simulink library "Ramp_Library_R2017b"  (R2017b)
settings: Solver=VariableStepAuto  StartTime=0.0  StopTime=10.0  RelTol=1e-3
libraries: simulink x52
(part 1 of 2)
Description:
  | VLS Standard Library
  | Version: 1.0.0
settings Model: Creator=mchawa  LastModifiedBy=mchawa

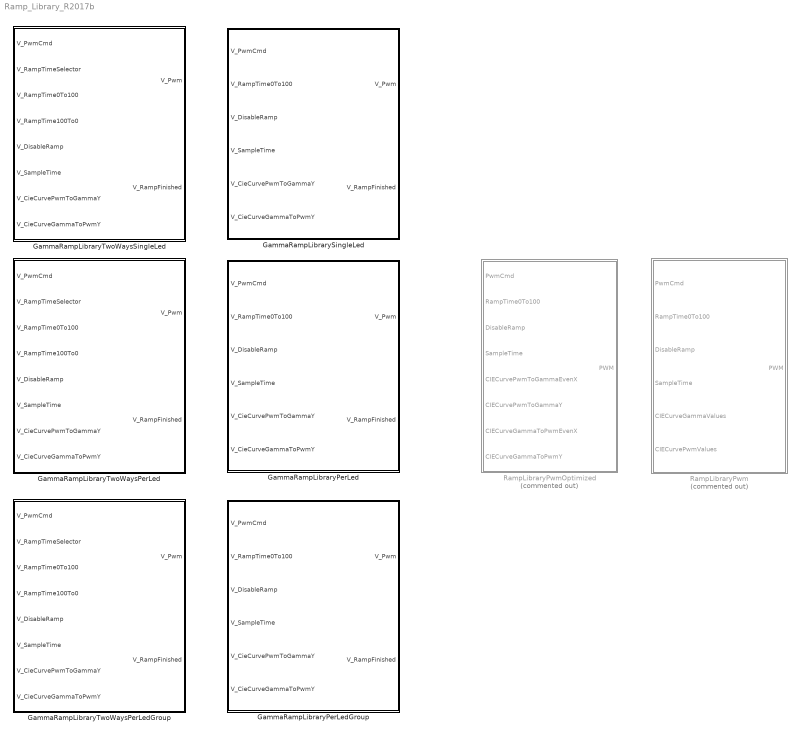
== system Ramp_Library_R2017b ==
  GammaRampLibraryPerLed : Subsystem  Description=|
      | This library performs ramp function taking CIE curves which are evenly distributed.
      | It performs the ramp linearly on the Gamma Curve.
  GammaRampLibraryPerLedGroup : Subsystem  Description=|
      | This library performs ramp function taking CIE curves which are evenly distributed.
      | It performs the ramp linearly on the Gamma Curve.
  GammaRampLibrarySingleLed : Subsystem  Description=|
      | This library performs ramp function taking CIE curves which are evenly distributed.
      | It performs the ramp linearly on the Gamma Curve.
  GammaRampLibraryTwoWaysPerLed : Subsystem  Description=|
      | This library performs ramp function taking CIE curves which are evenly distributed.
      | It performs the ramp linearly on the Gamma Curve.
  GammaRampLibraryTwoWaysPerLedGroup : Subsystem  Description=|
      | This library performs ramp function taking CIE curves which are evenly distributed.
      | It performs the ramp linearly on the Gamma Curve.
  GammaRampLibraryTwoWaysSingleLed : Subsystem  Description=|
      | This library performs ramp function taking CIE curves which are evenly distributed.
      | It performs the ramp linearly on the Gamma Curve.
  RampLibraryPwm : Subsystem  Description=|  Commented=on
      | This library performs ramp function taking CIE curves.
      | It performs the ramp linearly on the Pwm Curve.
  RampLibraryPwmOptimized : Subsystem  Description=|  Commented=on
      | This library performs ramp function taking CIE curves which are evenly distributed.
      | It performs the ramp linearly on the Pwm Curve.

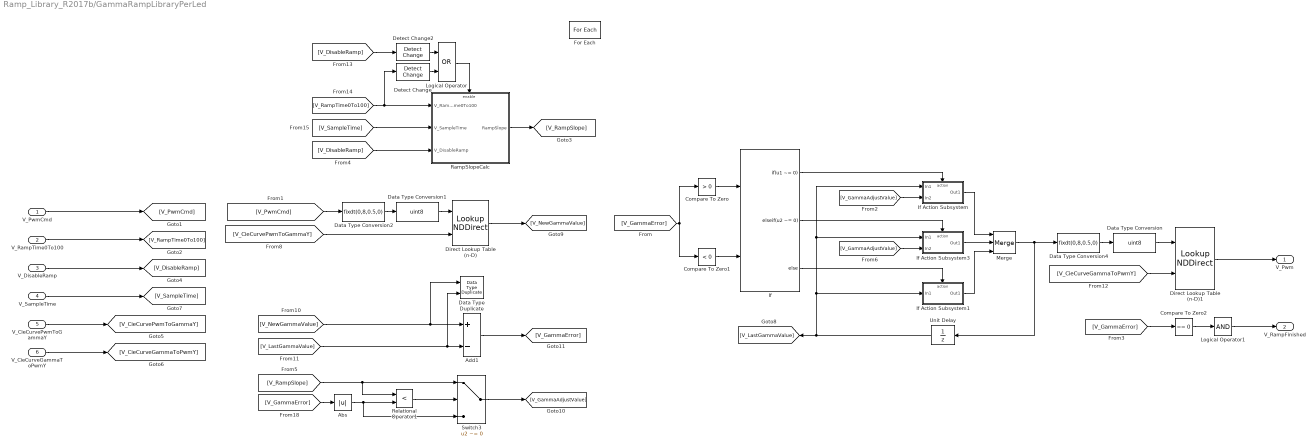
== system Ramp_Library_R2017b/GammaRampLibraryPerLed ==
  V_PwmCmd : Inport  Partition=on  PartitionDimension=1  PartitionWidth=1  PartitionOffset=0
  V_RampTime0To100 : Inport  Port=2  Partition=on  PartitionDimension=1  PartitionWidth=1  PartitionOffset=0
  V_DisableRamp : Inport  Port=3
  V_SampleTime : Inport  Port=4
  V_CieCurvePwmToGammaY : Inport  Port=5
  V_CieCurveGammaToPwmY : Inport  Port=6
  Abs : Abs
  Add1 : Sum  Inputs=+-  OutMin=-100  OutMax=100  OutDataTypeStr=fixdt(1,16,0.01,0)
  Compare To Zero : simulink/Logic and Bit Operations/Compare To Zero  relop=>  OutDataTypeStr=boolean
  Compare To Zero1 : simulink/Logic and Bit Operations/Compare To Zero  relop=<  OutDataTypeStr=boolean
  Compare To Zero2 : simulink/Logic and Bit Operations/Compare To Zero  relop===  OutDataTypeStr=boolean
  Data Type Duplicate : DataTypeDuplicate
  Data Type Conversion : DataTypeConversion  OutDataTypeStr=uint8  ConvertRealWorld=Stored Integer (SI)
  Data Type Conversion1 : DataTypeConversion  OutDataTypeStr=uint8  ConvertRealWorld=Stored Integer (SI)
  Data Type Conversion2 : DataTypeConversion  OutDataTypeStr=fixdt(0,8,0.5,0)  RndMeth=Round
  Data Type Conversion4 : DataTypeConversion  OutDataTypeStr=fixdt(0,8,0.5,0)  RndMeth=Round
  Detect Change : simulink/Logic and Bit Operations/Detect Change  vinit=0  OutDataTypeStr=boolean
  Detect Change2 : simulink/Logic and Bit Operations/Detect Change  vinit=0  OutDataTypeStr=boolean
  Direct Lookup Table (n-D) : LookupNDDirect  NumberOfTableDimensions=1  TableIsInput=on
  Direct Lookup Table (n-D)1 : LookupNDDirect  NumberOfTableDimensions=1  TableIsInput=on
  For Each : ForEach  DisableCoverage=on  IndexMode=One-based
  If : If  NumInputs=2  IfExpression=u1 ~= 0  ElseIfExpressions=u2 ~= 0
  If Action Subsystem : Subsystem  TreatAsAtomicUnit=on
  If Action Subsystem1 : Subsystem  TreatAsAtomicUnit=on
  If Action Subsystem3 : Subsystem  TreatAsAtomicUnit=on
  Logical Operator : Logic  Operator=OR  AllPortsSameDT=off  OutDataTypeStr=boolean
  Logical Operator1 : Logic  Inputs=1  AllPortsSameDT=off  OutDataTypeStr=boolean
  Merge : Merge  Inputs=3
  RampSlopeCalc : Subsystem  TreatAsAtomicUnit=on
  Relational Operator1 : RelationalOperator  Operator=<  OutDataTypeStr=boolean  RndMeth=Simplest
  Switch3 : Switch  Criteria=u2 ~= 0  OutDataTypeStr=Inherit: Inherit via back propagation
  Unit Delay : UnitDelay  SampleTime=-1
  V_Pwm : Outport  ConcatenationDimension=1
  V_RampFinished : Outport  Port=2  ConcatenationDimension=1
  wires:
  [V_CieCurveGammaToPwmY] -> Direct Lookup Table (n-D)1/2
  [V_GammaError] -> Compare To Zero1/1, Compare To Zero/1
  [V_NewGammaValue] -> Add1/1, Data Type Duplicate/1
  If Action Subsystem/1(Out1) -> Merge/1
  If Action Subsystem1/1(Out1) -> Merge/3
  Abs/1 -> Switch3/3, Relational Operator1/2
  V_PwmCmd/1 -> [V_PwmCmd]
  V_CieCurvePwmToGammaY/1 -> [V_CieCurvePwmToGammaY]
  [V_GammaError] -> Abs/1
  [V_PwmCmd] -> Data Type Conversion2/1
  Data Type Conversion/1 -> Direct Lookup Table (n-D)1/1
  Detect Change/1 -> Logical Operator/2
  Data Type Conversion4/1 -> Data Type Conversion/1
  [V_CieCurvePwmToGammaY] -> Direct Lookup Table (n-D)/2
  Switch3/1 -> [V_GammaAdjustValue]
  V_SampleTime/1 -> [V_SampleTime]
  Relational Operator1/1 -> Switch3/2
  V_RampTime0To100/1 -> [V_RampTime0To100]
  Compare To Zero/1 -> If/1
  If/3 -> If Action Subsystem1/Action
  Unit Delay/1 -> If Action Subsystem/1(In1), If Action Subsystem3/1(In1), If Action Subsystem1/1(In1), [V_LastGammaValue]
  [V_GammaAdjustValue] -> If Action Subsystem/2(In2)
  [V_RampSlope] -> Switch3/1, Relational Operator1/1
  [V_RampTime0To100] -> Detect Change/1, RampSlopeCalc/1(V_RampTime0To100)
  If/2 -> If Action Subsystem3/Action
  V_DisableRamp/1 -> [V_DisableRamp]
  Data Type Conversion1/1 -> Direct Lookup Table (n-D)/1
  [V_DisableRamp] -> RampSlopeCalc/3(V_DisableRamp)
  [V_LastGammaValue] -> Add1/2, Data Type Duplicate/2
  Add1/1 -> [V_GammaError]
  Logical Operator/1 -> RampSlopeCalc/Enable
  Merge/1 -> Data Type Conversion4/1, Unit Delay/1
  Direct Lookup Table (n-D)/1 -> [V_NewGammaValue]
  [V_SampleTime] -> RampSlopeCalc/2(V_SampleTime)
  Direct Lookup Table (n-D)1/1 -> V_Pwm/1
  V_CieCurveGammaToPwmY/1 -> [V_CieCurveGammaToPwmY]
  [V_DisableRamp] -> Detect Change2/1
  Compare To Zero1/1 -> If/2
  Data Type Conversion2/1 -> Data Type Conversion1/1
  If Action Subsystem3/1(Out1) -> Merge/2
  [V_GammaAdjustValue] -> If Action Subsystem3/2(In2)
  RampSlopeCalc/1(RampSlope) -> [V_RampSlope]
  Detect Change2/1 -> Logical Operator/1
  If/1 -> If Action Subsystem/Action
  [V_GammaError] -> Compare To Zero2/1
  Compare To Zero2/1 -> Logical Operator1/1
  Logical Operator1/1 -> V_RampFinished/1

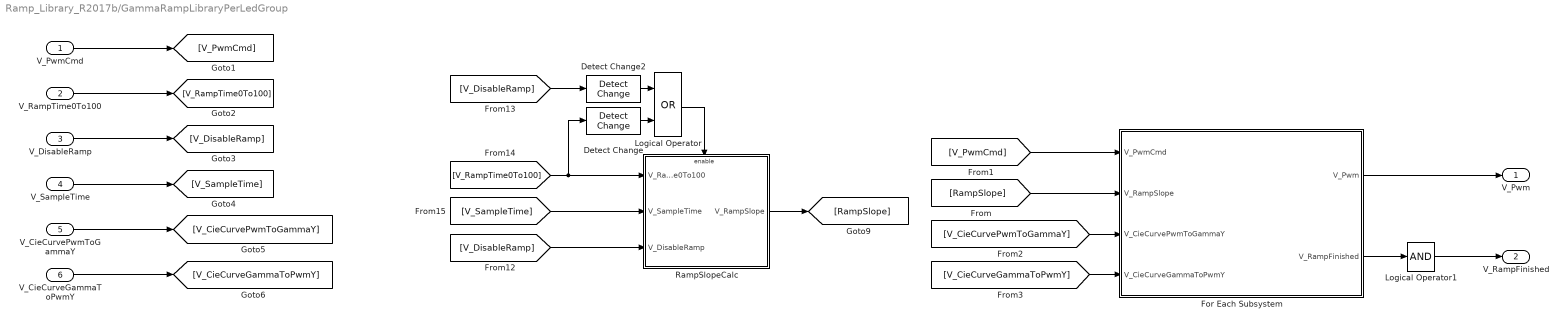
== system Ramp_Library_R2017b/GammaRampLibraryPerLedGroup ==
  V_PwmCmd : Inport
  V_RampTime0To100 : Inport  Port=2
  V_DisableRamp : Inport  Port=3
  V_SampleTime : Inport  Port=4
  V_CieCurvePwmToGammaY : Inport  Port=5
  V_CieCurveGammaToPwmY : Inport  Port=6
  Detect Change : simulink/Logic and Bit Operations/Detect Change  vinit=0  OutDataTypeStr=boolean
  Detect Change2 : simulink/Logic and Bit Operations/Detect Change  vinit=0  OutDataTypeStr=boolean
  For Each Subsystem : Subsystem  TreatAsAtomicUnit=on
  Logical Operator : Logic  Operator=OR  AllPortsSameDT=off  OutDataTypeStr=boolean
  Logical Operator1 : Logic  Inputs=1  AllPortsSameDT=off  OutDataTypeStr=boolean
  RampSlopeCalc : Subsystem  TreatAsAtomicUnit=on
  V_Pwm : Outport
  V_RampFinished : Outport  Port=2
  wires:
  V_PwmCmd/1 -> [V_PwmCmd]
  V_RampTime0To100/1 -> [V_RampTime0To100]
  V_DisableRamp/1 -> [V_DisableRamp]
  V_SampleTime/1 -> [V_SampleTime]
  V_CieCurvePwmToGammaY/1 -> [V_CieCurvePwmToGammaY]
  V_CieCurveGammaToPwmY/1 -> [V_CieCurveGammaToPwmY]
  RampSlopeCalc/1(V_RampSlope) -> [RampSlope]
  Logical Operator/1 -> RampSlopeCalc/Enable
  Detect Change/1 -> Logical Operator/2
  [V_DisableRamp] -> Detect Change2/1
  [V_DisableRamp] -> RampSlopeCalc/3(V_DisableRamp)
  [V_SampleTime] -> RampSlopeCalc/2(V_SampleTime)
  [V_RampTime0To100] -> RampSlopeCalc/1(V_RampTime0To100), Detect Change/1
  Detect Change2/1 -> Logical Operator/1
  [RampSlope] -> For Each Subsystem/2(V_RampSlope)
  [V_PwmCmd] -> For Each Subsystem/1(V_PwmCmd)
  [V_CieCurvePwmToGammaY] -> For Each Subsystem/3(V_CieCurvePwmToGammaY)
  For Each Subsystem/1(V_Pwm) -> V_Pwm/1
  [V_CieCurveGammaToPwmY] -> For Each Subsystem/4(V_CieCurveGammaToPwmY)
  For Each Subsystem/2(V_RampFinished) -> Logical Operator1/1
  Logical Operator1/1 -> V_RampFinished/1

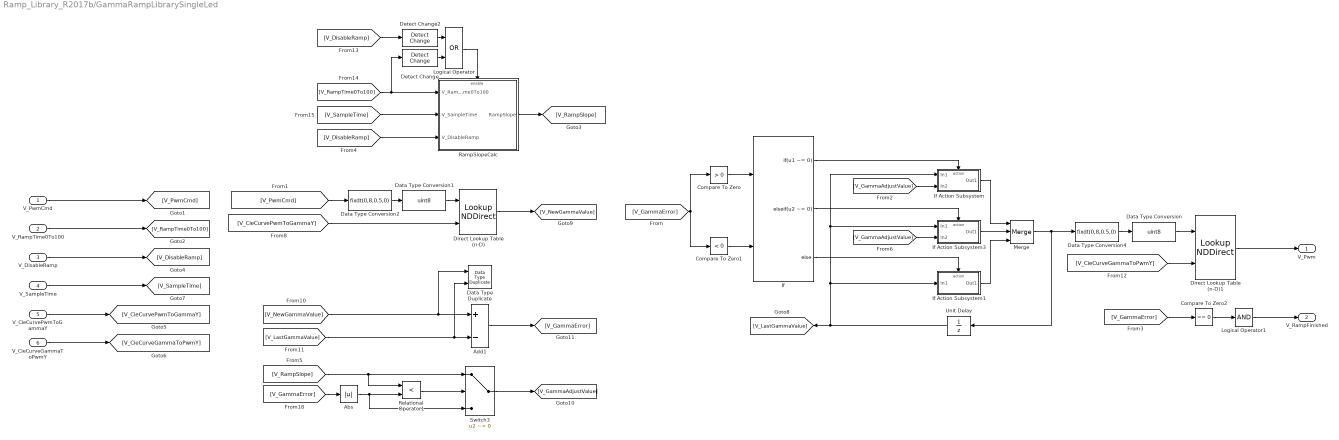
== system Ramp_Library_R2017b/GammaRampLibrarySingleLed ==
  V_PwmCmd : Inport
  V_RampTime0To100 : Inport  Port=2
  V_DisableRamp : Inport  Port=3
  V_SampleTime : Inport  Port=4
  V_CieCurvePwmToGammaY : Inport  Port=5
  V_CieCurveGammaToPwmY : Inport  Port=6
  Abs : Abs
  Add1 : Sum  Inputs=+-  OutMin=-100  OutMax=100  OutDataTypeStr=fixdt(1,16,0.01,0)
  Compare To Zero : simulink/Logic and Bit Operations/Compare To Zero  relop=>  OutDataTypeStr=boolean
  Compare To Zero1 : simulink/Logic and Bit Operations/Compare To Zero  relop=<  OutDataTypeStr=boolean
  Compare To Zero2 : simulink/Logic and Bit Operations/Compare To Zero  relop===  OutDataTypeStr=boolean
  Data Type Duplicate : DataTypeDuplicate
  Data Type Conversion : DataTypeConversion  OutDataTypeStr=uint8  ConvertRealWorld=Stored Integer (SI)
  Data Type Conversion1 : DataTypeConversion  OutDataTypeStr=uint8  ConvertRealWorld=Stored Integer (SI)
  Data Type Conversion2 : DataTypeConversion  OutDataTypeStr=fixdt(0,8,0.5,0)  RndMeth=Round
  Data Type Conversion4 : DataTypeConversion  OutDataTypeStr=fixdt(0,8,0.5,0)  RndMeth=Round
  Detect Change : simulink/Logic and Bit Operations/Detect Change  vinit=0  OutDataTypeStr=boolean
  Detect Change2 : simulink/Logic and Bit Operations/Detect Change  vinit=0  OutDataTypeStr=boolean
  Direct Lookup Table (n-D) : LookupNDDirect  NumberOfTableDimensions=1  TableIsInput=on
  Direct Lookup Table (n-D)1 : LookupNDDirect  NumberOfTableDimensions=1  TableIsInput=on
  If : If  NumInputs=2  IfExpression=u1 ~= 0  ElseIfExpressions=u2 ~= 0
  If Action Subsystem : Subsystem  TreatAsAtomicUnit=on
  If Action Subsystem1 : Subsystem  TreatAsAtomicUnit=on
  If Action Subsystem3 : Subsystem  TreatAsAtomicUnit=on
  Logical Operator : Logic  Operator=OR  AllPortsSameDT=off  OutDataTypeStr=boolean
  Logical Operator1 : Logic  Inputs=1  AllPortsSameDT=off  OutDataTypeStr=boolean
  Merge : Merge  Inputs=3
  RampSlopeCalc : Subsystem  TreatAsAtomicUnit=on
  Relational Operator1 : RelationalOperator  Operator=<  OutDataTypeStr=boolean  RndMeth=Simplest
  Switch3 : Switch  Criteria=u2 ~= 0  OutDataTypeStr=Inherit: Inherit via back propagation
  Unit Delay : UnitDelay  SampleTime=-1
  V_Pwm : Outport
  V_RampFinished : Outport  Port=2
  wires:
  Logical Operator1/1 -> V_RampFinished/1
  Compare To Zero2/1 -> Logical Operator1/1
  [V_GammaError] -> Compare To Zero2/1
  If/1 -> If Action Subsystem/Action
  Detect Change2/1 -> Logical Operator/1
  RampSlopeCalc/1(RampSlope) -> [V_RampSlope]
  [V_GammaAdjustValue] -> If Action Subsystem3/2(In2)
  If Action Subsystem3/1(Out1) -> Merge/2
  Data Type Conversion2/1 -> Data Type Conversion1/1
  Compare To Zero1/1 -> If/2
  [V_DisableRamp] -> Detect Change2/1
  V_CieCurveGammaToPwmY/1 -> [V_CieCurveGammaToPwmY]
  Direct Lookup Table (n-D)1/1 -> V_Pwm/1
  [V_SampleTime] -> RampSlopeCalc/2(V_SampleTime)
  Direct Lookup Table (n-D)/1 -> [V_NewGammaValue]
  Merge/1 -> Unit Delay/1, Data Type Conversion4/1
  Logical Operator/1 -> RampSlopeCalc/Enable
  Add1/1 -> [V_GammaError]
  [V_LastGammaValue] -> Data Type Duplicate/2, Add1/2
  [V_DisableRamp] -> RampSlopeCalc/3(V_DisableRamp)
  Data Type Conversion1/1 -> Direct Lookup Table (n-D)/1
  V_DisableRamp/1 -> [V_DisableRamp]
  If/2 -> If Action Subsystem3/Action
  [V_RampTime0To100] -> RampSlopeCalc/1(V_RampTime0To100), Detect Change/1
  [V_RampSlope] -> Relational Operator1/1, Switch3/1
  [V_GammaAdjustValue] -> If Action Subsystem/2(In2)
  Unit Delay/1 -> [V_LastGammaValue], If Action Subsystem1/1(In1), If Action Subsystem3/1(In1), If Action Subsystem/1(In1)
  If/3 -> If Action Subsystem1/Action
  Compare To Zero/1 -> If/1
  V_RampTime0To100/1 -> [V_RampTime0To100]
  Relational Operator1/1 -> Switch3/2
  V_SampleTime/1 -> [V_SampleTime]
  Switch3/1 -> [V_GammaAdjustValue]
  [V_CieCurvePwmToGammaY] -> Direct Lookup Table (n-D)/2
  Data Type Conversion4/1 -> Data Type Conversion/1
  Detect Change/1 -> Logical Operator/2
  Data Type Conversion/1 -> Direct Lookup Table (n-D)1/1
  [V_PwmCmd] -> Data Type Conversion2/1
  [V_GammaError] -> Abs/1
  V_CieCurvePwmToGammaY/1 -> [V_CieCurvePwmToGammaY]
  V_PwmCmd/1 -> [V_PwmCmd]
  Abs/1 -> Relational Operator1/2, Switch3/3
  If Action Subsystem1/1(Out1) -> Merge/3
  If Action Subsystem/1(Out1) -> Merge/1
  [V_NewGammaValue] -> Data Type Duplicate/1, Add1/1
  [V_GammaError] -> Compare To Zero/1, Compare To Zero1/1
  [V_CieCurveGammaToPwmY] -> Direct Lookup Table (n-D)1/2

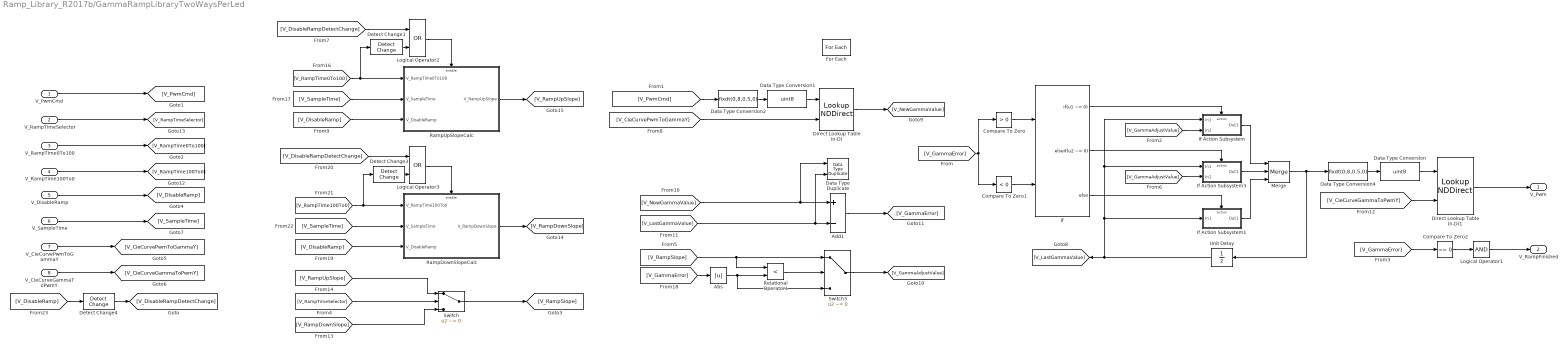
== system Ramp_Library_R2017b/GammaRampLibraryTwoWaysPerLed ==
  V_PwmCmd : Inport  Partition=on  PartitionDimension=1  PartitionWidth=1  PartitionOffset=0
  V_RampTimeSelector : Inport  Port=2  Partition=on  PartitionDimension=1  PartitionWidth=1  PartitionOffset=0
  V_RampTime0To100 : Inport  Port=3  Partition=on  PartitionDimension=1  PartitionWidth=1  PartitionOffset=0
  V_RampTime100To0 : Inport  Port=4  Partition=on  PartitionDimension=1  PartitionWidth=1  PartitionOffset=0
  V_DisableRamp : Inport  Port=5
  V_SampleTime : Inport  Port=6
  V_CieCurvePwmToGammaY : Inport  Port=7
  V_CieCurveGammaToPwmY : Inport  Port=8
  Abs : Abs
  Add1 : Sum  Inputs=+-  OutMin=-100  OutMax=100  OutDataTypeStr=fixdt(1,16,0.01,0)
  Compare To Zero : simulink/Logic and Bit Operations/Compare To Zero  relop=>  OutDataTypeStr=boolean
  Compare To Zero1 : simulink/Logic and Bit Operations/Compare To Zero  relop=<  OutDataTypeStr=boolean
  Compare To Zero2 : simulink/Logic and Bit Operations/Compare To Zero  relop===  OutDataTypeStr=boolean
  Data Type Duplicate : DataTypeDuplicate
  Data Type Conversion : DataTypeConversion  OutDataTypeStr=uint8  ConvertRealWorld=Stored Integer (SI)
  Data Type Conversion1 : DataTypeConversion  OutDataTypeStr=uint8  ConvertRealWorld=Stored Integer (SI)
  Data Type Conversion2 : DataTypeConversion  OutDataTypeStr=fixdt(0,8,0.5,0)  RndMeth=Round
  Data Type Conversion4 : DataTypeConversion  OutDataTypeStr=fixdt(0,8,0.5,0)  RndMeth=Round
  Detect Change1 : simulink/Logic and Bit Operations/Detect Change  vinit=0  OutDataTypeStr=boolean
  Detect Change3 : simulink/Logic and Bit Operations/Detect Change  vinit=0  OutDataTypeStr=boolean
  Detect Change4 : simulink/Logic and Bit Operations/Detect Change  vinit=0  OutDataTypeStr=boolean
  Direct Lookup Table (n-D) : LookupNDDirect  NumberOfTableDimensions=1  TableIsInput=on
  Direct Lookup Table (n-D)1 : LookupNDDirect  NumberOfTableDimensions=1  TableIsInput=on
  For Each : ForEach  DisableCoverage=on  IndexMode=One-based
  If : If  NumInputs=2  IfExpression=u1 ~= 0  ElseIfExpressions=u2 ~= 0
  If Action Subsystem : Subsystem  TreatAsAtomicUnit=on
  If Action Subsystem1 : Subsystem  TreatAsAtomicUnit=on
  If Action Subsystem3 : Subsystem  TreatAsAtomicUnit=on
  Logical Operator1 : Logic  Inputs=1  AllPortsSameDT=off  OutDataTypeStr=boolean
  Logical Operator2 : Logic  Operator=OR  AllPortsSameDT=off  OutDataTypeStr=boolean
  Logical Operator3 : Logic  Operator=OR  AllPortsSameDT=off  OutDataTypeStr=boolean
  Merge : Merge  Inputs=3
  RampDownSlopeCalc : Subsystem  TreatAsAtomicUnit=on
  RampUpSlopeCalc : Subsystem  TreatAsAtomicUnit=on
  Relational Operator1 : RelationalOperator  Operator=<  OutDataTypeStr=boolean  RndMeth=Simplest
  Switch : Switch  Criteria=u2 ~= 0
  Switch3 : Switch  Criteria=u2 ~= 0  OutDataTypeStr=Inherit: Inherit via back propagation
  Unit Delay : UnitDelay  SampleTime=-1
  V_Pwm : Outport  ConcatenationDimension=1
  V_RampFinished : Outport  Port=2  ConcatenationDimension=1
  wires:
  Logical Operator1/1 -> V_RampFinished/1
  Compare To Zero2/1 -> Logical Operator1/1
  [V_GammaError] -> Compare To Zero2/1
  If/1 -> If Action Subsystem/Action
  [V_GammaAdjustValue] -> If Action Subsystem3/2(In2)
  If Action Subsystem3/1(Out1) -> Merge/2
  Data Type Conversion2/1 -> Data Type Conversion1/1
  Compare To Zero1/1 -> If/2
  V_CieCurveGammaToPwmY/1 -> [V_CieCurveGammaToPwmY]
  Direct Lookup Table (n-D)1/1 -> V_Pwm/1
  Direct Lookup Table (n-D)/1 -> [V_NewGammaValue]
  Merge/1 -> Unit Delay/1, Data Type Conversion4/1
  Add1/1 -> [V_GammaError]
  [V_LastGammaValue] -> Data Type Duplicate/2, Add1/2
  Data Type Conversion1/1 -> Direct Lookup Table (n-D)/1
  V_DisableRamp/1 -> [V_DisableRamp]
  If/2 -> If Action Subsystem3/Action
  [V_RampSlope] -> Relational Operator1/1, Switch3/1
  [V_GammaAdjustValue] -> If Action Subsystem/2(In2)
  Unit Delay/1 -> [V_LastGammaValue], If Action Subsystem1/1(In1), If Action Subsystem3/1(In1), If Action Subsystem/1(In1)
  If/3 -> If Action Subsystem1/Action
  Compare To Zero/1 -> If/1
  V_RampTime0To100/1 -> [V_RampTime0To100]
  Relational Operator1/1 -> Switch3/2
  V_SampleTime/1 -> [V_SampleTime]
  Switch3/1 -> [V_GammaAdjustValue]
  [V_CieCurvePwmToGammaY] -> Direct Lookup Table (n-D)/2
  Data Type Conversion4/1 -> Data Type Conversion/1
  Data Type Conversion/1 -> Direct Lookup Table (n-D)1/1
  [V_PwmCmd] -> Data Type Conversion2/1
  [V_GammaError] -> Abs/1
  V_CieCurvePwmToGammaY/1 -> [V_CieCurvePwmToGammaY]
  V_PwmCmd/1 -> [V_PwmCmd]
  Abs/1 -> Relational Operator1/2, Switch3/3
  If Action Subsystem1/1(Out1) -> Merge/3
  If Action Subsystem/1(Out1) -> Merge/1
  [V_NewGammaValue] -> Data Type Duplicate/1, Add1/1
  [V_GammaError] -> Compare To Zero1/1, Compare To Zero/1
  [V_CieCurveGammaToPwmY] -> Direct Lookup Table (n-D)1/2
  V_RampTime100To0/1 -> [V_RampTime100To0]
  V_RampTimeSelector/1 -> [V_RampTimeSelector]
  Logical Operator2/1 -> RampUpSlopeCalc/Enable
  Detect Change3/1 -> Logical Operator3/2
  RampDownSlopeCalc/1(V_RampDownSlope) -> [V_RampDownSlope]
  [V_SampleTime] -> RampUpSlopeCalc/2(V_SampleTime)
  [V_DisableRampDetectChange] -> Logical Operator2/1
  [V_DisableRampDetectChange] -> Logical Operator3/1
  RampUpSlopeCalc/1(V_RampUpSlope) -> [V_RampUpSlope]
  Detect Change1/1 -> Logical Operator2/2
  [V_DisableRamp] -> RampDownSlopeCalc/3(V_DisableRamp)
  [V_RampTime100To0] -> RampDownSlopeCalc/1(V_RampTime100To0), Detect Change3/1
  [V_SampleTime] -> RampDownSlopeCalc/2(V_SampleTime)
  [V_DisableRamp] -> RampUpSlopeCalc/3(V_DisableRamp)
  Logical Operator3/1 -> RampDownSlopeCalc/Enable
  [V_RampTime0To100] -> Detect Change1/1, RampUpSlopeCalc/1(V_RampTime0To100)
  [V_DisableRamp] -> Detect Change4/1
  Detect Change4/1 -> [V_DisableRampDetectChange]
  [V_RampDownSlope] -> Switch/3
  [V_RampTimeSelector] -> Switch/2
  Switch/1 -> [V_RampSlope]
  [V_RampUpSlope] -> Switch/1

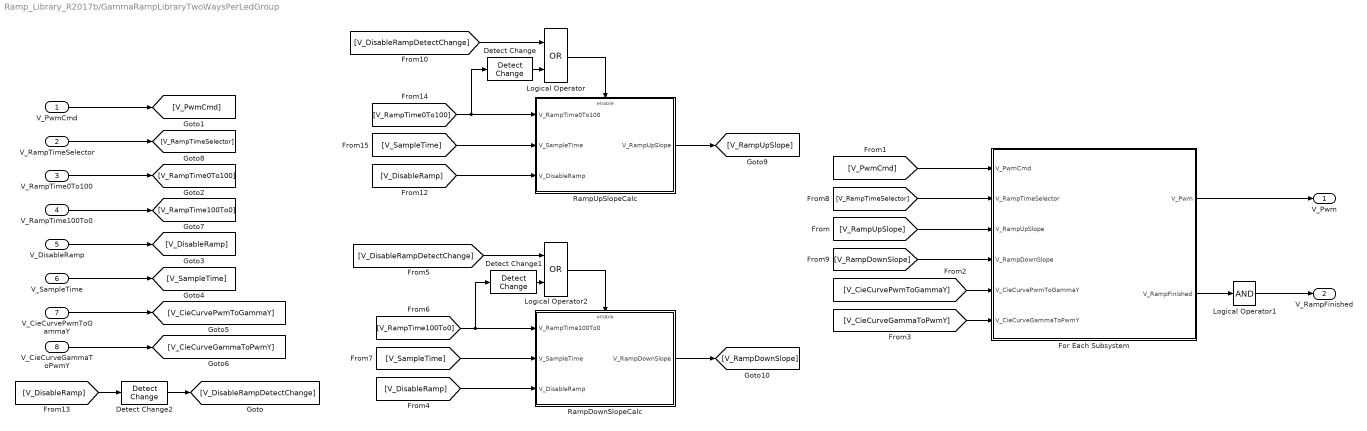
== system Ramp_Library_R2017b/GammaRampLibraryTwoWaysPerLedGroup ==
  V_PwmCmd : Inport
  V_RampTimeSelector : Inport  Port=2
  V_RampTime0To100 : Inport  Port=3
  V_RampTime100To0 : Inport  Port=4
  V_DisableRamp : Inport  Port=5
  V_SampleTime : Inport  Port=6
  V_CieCurvePwmToGammaY : Inport  Port=7
  V_CieCurveGammaToPwmY : Inport  Port=8
  Detect Change : simulink/Logic and Bit Operations/Detect Change  vinit=0  OutDataTypeStr=boolean
  Detect Change1 : simulink/Logic and Bit Operations/Detect Change  vinit=0  OutDataTypeStr=boolean
  Detect Change2 : simulink/Logic and Bit Operations/Detect Change  vinit=0  OutDataTypeStr=boolean
  For Each Subsystem : Subsystem  TreatAsAtomicUnit=on
  Logical Operator : Logic  Operator=OR  AllPortsSameDT=off  OutDataTypeStr=boolean
  Logical Operator1 : Logic  Inputs=1  AllPortsSameDT=off  OutDataTypeStr=boolean
  Logical Operator2 : Logic  Operator=OR  AllPortsSameDT=off  OutDataTypeStr=boolean
  RampDownSlopeCalc : Subsystem  TreatAsAtomicUnit=on
  RampUpSlopeCalc : Subsystem  TreatAsAtomicUnit=on
  V_Pwm : Outport
  V_RampFinished : Outport  Port=2
  wires:
  Logical Operator1/1 -> V_RampFinished/1
  For Each Subsystem/2(V_RampFinished) -> Logical Operator1/1
  [V_CieCurveGammaToPwmY] -> For Each Subsystem/6(V_CieCurveGammaToPwmY)
  For Each Subsystem/1(V_Pwm) -> V_Pwm/1
  [V_CieCurvePwmToGammaY] -> For Each Subsystem/5(V_CieCurvePwmToGammaY)
  [V_PwmCmd] -> For Each Subsystem/1(V_PwmCmd)
  [V_RampUpSlope] -> For Each Subsystem/3(V_RampUpSlope)
  [V_RampTime0To100] -> Detect Change/1, RampUpSlopeCalc/1(V_RampTime0To100)
  [V_SampleTime] -> RampUpSlopeCalc/2(V_SampleTime)
  [V_DisableRamp] -> RampUpSlopeCalc/3(V_DisableRamp)
  [V_DisableRamp] -> Detect Change2/1
  Detect Change/1 -> Logical Operator/2
  Logical Operator/1 -> RampUpSlopeCalc/Enable
  RampUpSlopeCalc/1(V_RampUpSlope) -> [V_RampUpSlope]
  V_CieCurveGammaToPwmY/1 -> [V_CieCurveGammaToPwmY]
  V_CieCurvePwmToGammaY/1 -> [V_CieCurvePwmToGammaY]
  V_SampleTime/1 -> [V_SampleTime]
  V_DisableRamp/1 -> [V_DisableRamp]
  V_RampTime0To100/1 -> [V_RampTime0To100]
  V_PwmCmd/1 -> [V_PwmCmd]
  V_RampTime100To0/1 -> [V_RampTime100To0]
  V_RampTimeSelector/1 -> [V_RampTimeSelector]
  [V_DisableRamp] -> RampDownSlopeCalc/3(V_DisableRamp)
  [V_SampleTime] -> RampDownSlopeCalc/2(V_SampleTime)
  [V_RampTime100To0] -> RampDownSlopeCalc/1(V_RampTime100To0), Detect Change1/1
  Logical Operator2/1 -> RampDownSlopeCalc/Enable
  [V_DisableRampDetectChange] -> Logical Operator2/1
  Detect Change1/1 -> Logical Operator2/2
  RampDownSlopeCalc/1(V_RampDownSlope) -> [V_RampDownSlope]
  [V_RampTimeSelector] -> For Each Subsystem/2(V_RampTimeSelector)
  [V_RampDownSlope] -> For Each Subsystem/4(V_RampDownSlope)
  Detect Change2/1 -> [V_DisableRampDetectChange]
  [V_DisableRampDetectChange] -> Logical Operator/1

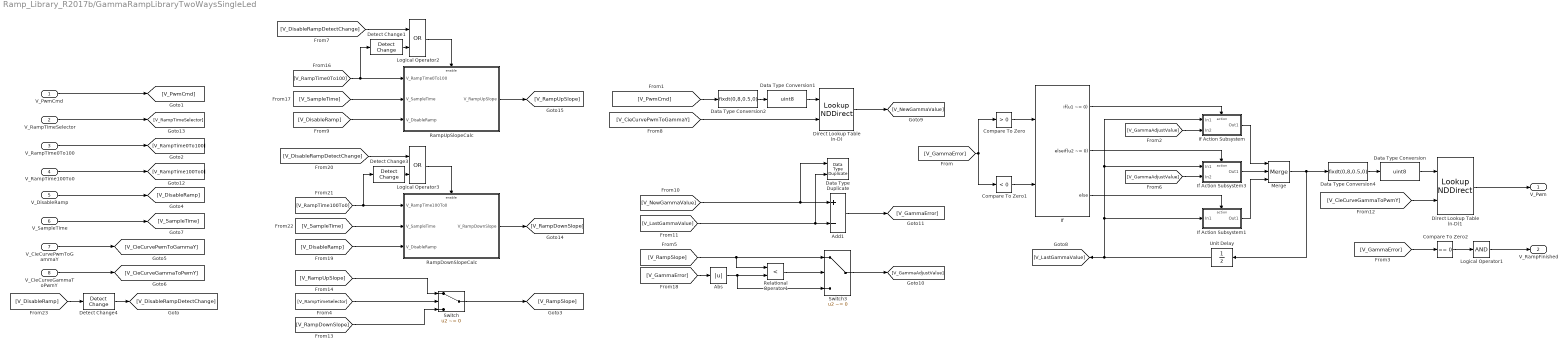
== system Ramp_Library_R2017b/GammaRampLibraryTwoWaysSingleLed ==
  V_PwmCmd : Inport
  V_RampTimeSelector : Inport  Port=2
  V_RampTime0To100 : Inport  Port=3
  V_RampTime100To0 : Inport  Port=4
  V_DisableRamp : Inport  Port=5
  V_SampleTime : Inport  Port=6
  V_CieCurvePwmToGammaY : Inport  Port=7
  V_CieCurveGammaToPwmY : Inport  Port=8
  Abs : Abs
  Add1 : Sum  Inputs=+-  OutMin=-100  OutMax=100  OutDataTypeStr=fixdt(1,16,0.01,0)
  Compare To Zero : simulink/Logic and Bit Operations/Compare To Zero  relop=>  OutDataTypeStr=boolean
  Compare To Zero1 : simulink/Logic and Bit Operations/Compare To Zero  relop=<  OutDataTypeStr=boolean
  Compare To Zero2 : simulink/Logic and Bit Operations/Compare To Zero  relop===  OutDataTypeStr=boolean
  Data Type Duplicate : DataTypeDuplicate
  Data Type Conversion : DataTypeConversion  OutDataTypeStr=uint8  ConvertRealWorld=Stored Integer (SI)
  Data Type Conversion1 : DataTypeConversion  OutDataTypeStr=uint8  ConvertRealWorld=Stored Integer (SI)
  Data Type Conversion2 : DataTypeConversion  OutDataTypeStr=fixdt(0,8,0.5,0)  RndMeth=Round
  Data Type Conversion4 : DataTypeConversion  OutDataTypeStr=fixdt(0,8,0.5,0)  RndMeth=Round
  Detect Change1 : simulink/Logic and Bit Operations/Detect Change  vinit=0  OutDataTypeStr=boolean
  Detect Change3 : simulink/Logic and Bit Operations/Detect Change  vinit=0  OutDataTypeStr=boolean
  Detect Change4 : simulink/Logic and Bit Operations/Detect Change  vinit=0  OutDataTypeStr=boolean
  Direct Lookup Table (n-D) : LookupNDDirect  NumberOfTableDimensions=1  TableIsInput=on
  Direct Lookup Table (n-D)1 : LookupNDDirect  NumberOfTableDimensions=1  TableIsInput=on
  If : If  NumInputs=2  IfExpression=u1 ~= 0  ElseIfExpressions=u2 ~= 0
  If Action Subsystem : Subsystem  TreatAsAtomicUnit=on
  If Action Subsystem1 : Subsystem  TreatAsAtomicUnit=on
  If Action Subsystem3 : Subsystem  TreatAsAtomicUnit=on
  Logical Operator1 : Logic  Inputs=1  AllPortsSameDT=off  OutDataTypeStr=boolean
  Logical Operator2 : Logic  Operator=OR  AllPortsSameDT=off  OutDataTypeStr=boolean
  Logical Operator3 : Logic  Operator=OR  AllPortsSameDT=off  OutDataTypeStr=boolean
  Merge : Merge  Inputs=3
  RampDownSlopeCalc : Subsystem  TreatAsAtomicUnit=on
  RampUpSlopeCalc : Subsystem  TreatAsAtomicUnit=on
  Relational Operator1 : RelationalOperator  Operator=<  OutDataTypeStr=boolean  RndMeth=Simplest
  Switch : Switch  Criteria=u2 ~= 0
  Switch3 : Switch  Criteria=u2 ~= 0  OutDataTypeStr=Inherit: Inherit via back propagation
  Unit Delay : UnitDelay  SampleTime=-1
  V_Pwm : Outport
  V_RampFinished : Outport  Port=2
  wires:
  [V_RampUpSlope] -> Switch/1
  Switch/1 -> [V_RampSlope]
  [V_RampTimeSelector] -> Switch/2
  [V_RampDownSlope] -> Switch/3
  Detect Change4/1 -> [V_DisableRampDetectChange]
  [V_DisableRamp] -> Detect Change4/1
  [V_RampTime0To100] -> RampUpSlopeCalc/1(V_RampTime0To100), Detect Change1/1
  Logical Operator3/1 -> RampDownSlopeCalc/Enable
  [V_DisableRamp] -> RampUpSlopeCalc/3(V_DisableRamp)
  [V_SampleTime] -> RampDownSlopeCalc/2(V_SampleTime)
  [V_RampTime100To0] -> Detect Change3/1, RampDownSlopeCalc/1(V_RampTime100To0)
  [V_DisableRamp] -> RampDownSlopeCalc/3(V_DisableRamp)
  Detect Change1/1 -> Logical Operator2/2
  RampUpSlopeCalc/1(V_RampUpSlope) -> [V_RampUpSlope]
  [V_DisableRampDetectChange] -> Logical Operator3/1
  [V_DisableRampDetectChange] -> Logical Operator2/1
  [V_SampleTime] -> RampUpSlopeCalc/2(V_SampleTime)
  RampDownSlopeCalc/1(V_RampDownSlope) -> [V_RampDownSlope]
  Detect Change3/1 -> Logical Operator3/2
  Logical Operator2/1 -> RampUpSlopeCalc/Enable
  V_RampTimeSelector/1 -> [V_RampTimeSelector]
  V_RampTime100To0/1 -> [V_RampTime100To0]
  [V_CieCurveGammaToPwmY] -> Direct Lookup Table (n-D)1/2
  [V_GammaError] -> Compare To Zero/1, Compare To Zero1/1
  [V_NewGammaValue] -> Add1/1, Data Type Duplicate/1
  If Action Subsystem/1(Out1) -> Merge/1
  If Action Subsystem1/1(Out1) -> Merge/3
  Abs/1 -> Switch3/3, Relational Operator1/2
  V_PwmCmd/1 -> [V_PwmCmd]
  V_CieCurvePwmToGammaY/1 -> [V_CieCurvePwmToGammaY]
  [V_GammaError] -> Abs/1
  [V_PwmCmd] -> Data Type Conversion2/1
  Data Type Conversion/1 -> Direct Lookup Table (n-D)1/1
  Data Type Conversion4/1 -> Data Type Conversion/1
  [V_CieCurvePwmToGammaY] -> Direct Lookup Table (n-D)/2
  Switch3/1 -> [V_GammaAdjustValue]
  V_SampleTime/1 -> [V_SampleTime]
  Relational Operator1/1 -> Switch3/2
  V_RampTime0To100/1 -> [V_RampTime0To100]
  Compare To Zero/1 -> If/1
  If/3 -> If Action Subsystem1/Action
  Unit Delay/1 -> If Action Subsystem/1(In1), If Action Subsystem3/1(In1), If Action Subsystem1/1(In1), [V_LastGammaValue]
  [V_GammaAdjustValue] -> If Action Subsystem/2(In2)
  [V_RampSlope] -> Switch3/1, Relational Operator1/1
  If/2 -> If Action Subsystem3/Action
  V_DisableRamp/1 -> [V_DisableRamp]
  Data Type Conversion1/1 -> Direct Lookup Table (n-D)/1
  [V_LastGammaValue] -> Add1/2, Data Type Duplicate/2
  Add1/1 -> [V_GammaError]
  Merge/1 -> Data Type Conversion4/1, Unit Delay/1
  Direct Lookup Table (n-D)/1 -> [V_NewGammaValue]
  Direct Lookup Table (n-D)1/1 -> V_Pwm/1
  V_CieCurveGammaToPwmY/1 -> [V_CieCurveGammaToPwmY]
  Compare To Zero1/1 -> If/2
  Data Type Conversion2/1 -> Data Type Conversion1/1
  If Action Subsystem3/1(Out1) -> Merge/2
  [V_GammaAdjustValue] -> If Action Subsystem3/2(In2)
  If/1 -> If Action Subsystem/Action
  [V_GammaError] -> Compare To Zero2/1
  Compare To Zero2/1 -> Logical Operator1/1
  Logical Operator1/1 -> V_RampFinished/1

== system Ramp_Library_R2017b/RampLibraryPwm ==
  PwmCmd : Inport
  RampTime0To100 : Inport  Port=2
  DisableRamp : Inport  Port=3
  SampleTime : Inport  Port=4
  CIECurveGammaValues : Inport  Port=5
  CIECurvePwmValues : Inport  Port=6
  If1 : If  IfExpression=u1 ~= 0
  Merge1 : Merge  InitialOutput=0
  Relational Operator1 : RelationalOperator  Operator=~=  OutDataTypeStr=boolean  RndMeth=Simplest
  Subsystem : Subsystem
  Subsystem1 : Subsystem
  Unit Delay1 : UnitDelay  SampleTime=-1
  PWM : Outport
  wires:
  Subsystem/1(NewPWM) -> Merge1/2
  Subsystem1/1(NewPWM) -> Merge1/1
  [SampleTime] -> Subsystem1/4(SampleTime)
  [DisableRamp] -> Subsystem1/3(DisableRamp)
  [RampTime0To100] -> Subsystem1/2(RampTime0To100)
  [PwmCmd] -> Subsystem1/1(PwmCmd)
  [PwmCmd] -> Relational Operator1/1
  SampleTime/1 -> [SampleTime]
  DisableRamp/1 -> [DisableRamp]
  RampTime0To100/1 -> [RampTime0To100]
  PwmCmd/1 -> [PwmCmd]
  Merge1/1 -> PWM/1, Unit Delay1/1
  Unit Delay1/1 -> [PreviousPWM]
  [PreviousPWM] -> Subsystem/1(LastPWM)
  [PreviousPWM] -> Relational Operator1/2
  If1/1 -> Subsystem1/Action
  Relational Operator1/1 -> If1/1
  If1/2 -> Subsystem/Action
  CIECurveGammaValues/1 -> [CIECurveGammaValues]
  CIECurvePwmValues/1 -> [CIECurvePwmValues]
  [CIECurveGammaValues] -> Subsystem1/5(CIECurveGammaValues)
  [CIECurvePwmValues] -> Subsystem1/6(CIECurvePwmValues)

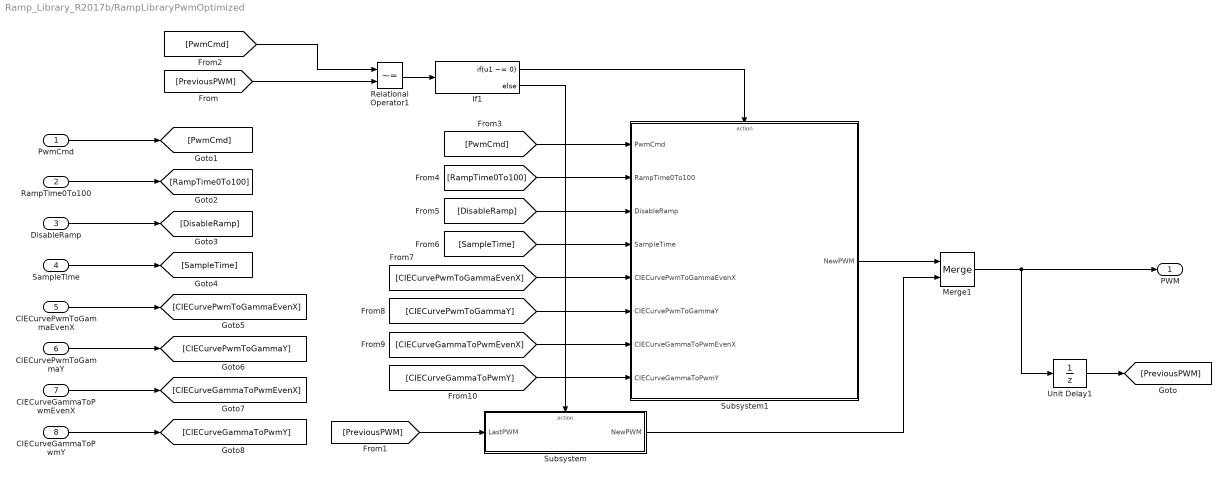
== system Ramp_Library_R2017b/RampLibraryPwmOptimized ==
  PwmCmd : Inport
  RampTime0To100 : Inport  Port=2
  DisableRamp : Inport  Port=3
  SampleTime : Inport  Port=4
  CIECurvePwmToGammaEvenX : Inport  Port=5
  CIECurvePwmToGammaY : Inport  Port=6
  CIECurveGammaToPwmEvenX : Inport  Port=7
  CIECurveGammaToPwmY : Inport  Port=8
  If1 : If  IfExpression=u1 ~= 0
  Merge1 : Merge  InitialOutput=0
  Relational Operator1 : RelationalOperator  Operator=~=  OutDataTypeStr=boolean  RndMeth=Simplest
  Subsystem : Subsystem
  Subsystem1 : Subsystem
  Unit Delay1 : UnitDelay  SampleTime=-1
  PWM : Outport
  wires:
  Subsystem/1(NewPWM) -> Merge1/2
  Subsystem1/1(NewPWM) -> Merge1/1
  [SampleTime] -> Subsystem1/4(SampleTime)
  [DisableRamp] -> Subsystem1/3(DisableRamp)
  [RampTime0To100] -> Subsystem1/2(RampTime0To100)
  [PwmCmd] -> Subsystem1/1(PwmCmd)
  [PwmCmd] -> Relational Operator1/1
  SampleTime/1 -> [SampleTime]
  DisableRamp/1 -> [DisableRamp]
  RampTime0To100/1 -> [RampTime0To100]
  PwmCmd/1 -> [PwmCmd]
  Merge1/1 -> PWM/1, Unit Delay1/1
  Unit Delay1/1 -> [PreviousPWM]
  [PreviousPWM] -> Subsystem/1(LastPWM)
  [PreviousPWM] -> Relational Operator1/2
  If1/1 -> Subsystem1/Action
  Relational Operator1/1 -> If1/1
  If1/2 -> Subsystem/Action
  CIECurveGammaToPwmEvenX/1 -> [CIECurveGammaToPwmEvenX]
  CIECurvePwmToGammaEvenX/1 -> [CIECurvePwmToGammaEvenX]
  CIECurveGammaToPwmY/1 -> [CIECurveGammaToPwmY]
  CIECurvePwmToGammaY/1 -> [CIECurvePwmToGammaY]
  [CIECurvePwmToGammaEvenX] -> Subsystem1/5(CIECurvePwmToGammaEvenX)
  [CIECurvePwmToGammaY] -> Subsystem1/6(CIECurvePwmToGammaY)
  [CIECurveGammaToPwmEvenX] -> Subsystem1/7(CIECurveGammaToPwmEvenX)
  [CIECurveGammaToPwmY] -> Subsystem1/8(CIECurveGammaToPwmY)

== system Ramp_Library_R2017b/GammaRampLibraryPerLed/If Action Subsystem ==
  In1 : Inport
  In2 : Inport  Port=2
  Action Port : ActionPort  ActionType=then
  Add : Sum  OutDataTypeStr=Inherit: Inherit via back propagation
  Out1 : Outport
  wires:
  In2/1 -> Add/2
  In1/1 -> Add/1
  Add/1 -> Out1/1

== system Ramp_Library_R2017b/GammaRampLibraryPerLed/If Action Subsystem1 ==
  In1 : Inport
  Action Port : ActionPort  ActionType=else
  Out1 : Outport
  wires:
  In1/1 -> Out1/1

== system Ramp_Library_R2017b/GammaRampLibraryPerLed/If Action Subsystem3 ==
  In1 : Inport
  In2 : Inport  Port=2
  Action Port : ActionPort  ActionType=elseif
  Add : Sum  Inputs=+-  OutDataTypeStr=Inherit: Inherit via back propagation
  Out1 : Outport
  wires:
  In2/1 -> Add/2
  In1/1 -> Add/1
  Add/1 -> Out1/1

== system Ramp_Library_R2017b/GammaRampLibraryPerLed/RampSlopeCalc ==
  V_RampTime0To100 : Inport
  V_SampleTime : Inport  Port=2
  V_DisableRamp : Inport  Port=3
  Enable : EnablePort
  Compare To Zero : simulink/Logic and Bit Operations/Compare To Zero  relop=~=  OutDataTypeStr=boolean
  Constant : Constant  Value=100  OutMin=0  OutMax=100  OutDataTypeStr=fixdt(0,16,0.01,0)
  If : If  IfExpression=u1 ~= 0
  If Action Subsystem : Subsystem  TreatAsAtomicUnit=on
  If Action Subsystem1 : Subsystem  TreatAsAtomicUnit=on
  Logical Operator : Logic  AllPortsSameDT=off  OutDataTypeStr=boolean
  Logical Operator1 : Logic  Operator=NOT  AllPortsSameDT=off  OutDataTypeStr=boolean
  Merge : Merge  InitialOutput=100
  RampSlope : Outport
  wires:
  If/1 -> If Action Subsystem/Action
  V_RampTime0To100/1 -> If Action Subsystem/2(Denominator), Compare To Zero/1
  Constant/1 -> If Action Subsystem1/1(DefaultValue)
  Merge/1 -> RampSlope/1
  If Action Subsystem/1(Result) -> Merge/1
  If Action Subsystem1/1(Result) -> Merge/2
  If/2 -> If Action Subsystem1/Action
  V_SampleTime/1 -> If Action Subsystem/1(Numerator)
  Compare To Zero/1 -> Logical Operator/1
  Logical Operator/1 -> If/1
  V_DisableRamp/1 -> Logical Operator1/1
  Logical Operator1/1 -> Logical Operator/2

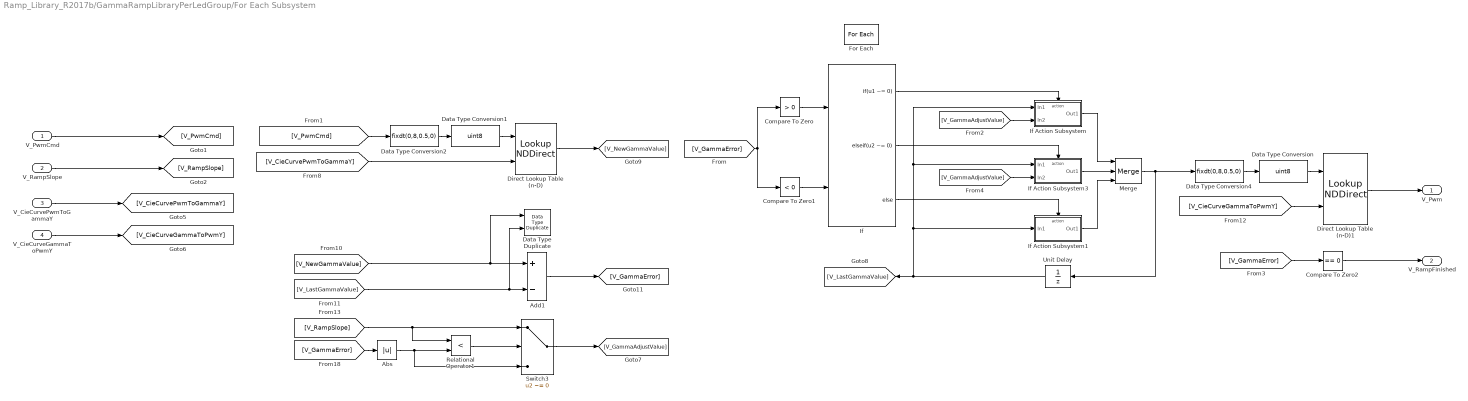
== system Ramp_Library_R2017b/GammaRampLibraryPerLedGroup/For Each Subsystem ==
  V_PwmCmd : Inport  Partition=on  PartitionDimension=1  PartitionWidth=1  PartitionOffset=0
  V_RampSlope : Inport  Port=2
  V_CieCurvePwmToGammaY : Inport  Port=3
  V_CieCurveGammaToPwmY : Inport  Port=4
  Abs : Abs
  Add1 : Sum  Inputs=+-  OutMin=-100  OutMax=100  OutDataTypeStr=fixdt(1,16,0.01,0)
  Compare To Zero : simulink/Logic and Bit Operations/Compare To Zero  relop=>  OutDataTypeStr=boolean
  Compare To Zero1 : simulink/Logic and Bit Operations/Compare To Zero  relop=<  OutDataTypeStr=boolean
  Compare To Zero2 : simulink/Logic and Bit Operations/Compare To Zero  relop===  OutDataTypeStr=boolean
  Data Type Duplicate : DataTypeDuplicate
  Data Type Conversion : DataTypeConversion  OutDataTypeStr=uint8  ConvertRealWorld=Stored Integer (SI)
  Data Type Conversion1 : DataTypeConversion  OutDataTypeStr=uint8  ConvertRealWorld=Stored Integer (SI)
  Data Type Conversion2 : DataTypeConversion  OutDataTypeStr=fixdt(0,8,0.5,0)  RndMeth=Round
  Data Type Conversion4 : DataTypeConversion  OutDataTypeStr=fixdt(0,8,0.5,0)  RndMeth=Round
  Direct Lookup Table (n-D) : LookupNDDirect  NumberOfTableDimensions=1  TableIsInput=on
  Direct Lookup Table (n-D)1 : LookupNDDirect  NumberOfTableDimensions=1  TableIsInput=on
  For Each : ForEach  DisableCoverage=on  IndexMode=One-based
  If : If  NumInputs=2  IfExpression=u1 ~= 0  ElseIfExpressions=u2 ~= 0
  If Action Subsystem : Subsystem  TreatAsAtomicUnit=on
  If Action Subsystem1 : Subsystem  TreatAsAtomicUnit=on
  If Action Subsystem3 : Subsystem  TreatAsAtomicUnit=on
  Merge : Merge  Inputs=3
  Relational Operator1 : RelationalOperator  Operator=<  OutDataTypeStr=boolean  RndMeth=Simplest
  Switch3 : Switch  Criteria=u2 ~= 0  OutDataTypeStr=Inherit: Inherit via back propagation
  Unit Delay : UnitDelay  SampleTime=-1
  V_Pwm : Outport  ConcatenationDimension=1
  V_RampFinished : Outport  Port=2  ConcatenationDimension=1
  wires:
  [V_PwmCmd] -> Data Type Conversion2/1
  Direct Lookup Table (n-D)/1 -> [V_NewGammaValue]
  V_PwmCmd/1 -> [V_PwmCmd]
  V_CieCurveGammaToPwmY/1 -> [V_CieCurveGammaToPwmY]
  V_CieCurvePwmToGammaY/1 -> [V_CieCurvePwmToGammaY]
  V_RampSlope/1 -> [V_RampSlope]
  Data Type Conversion2/1 -> Data Type Conversion1/1
  [V_CieCurvePwmToGammaY] -> Direct Lookup Table (n-D)/2
  Direct Lookup Table (n-D)1/1 -> V_Pwm/1
  [V_NewGammaValue] -> Data Type Duplicate/1, Add1/1
  [V_LastGammaValue] -> Data Type Duplicate/2, Add1/2
  [V_CieCurveGammaToPwmY] -> Direct Lookup Table (n-D)1/2
  Merge/1 -> Data Type Conversion4/1, Unit Delay/1
  Data Type Conversion1/1 -> Direct Lookup Table (n-D)/1
  Compare To Zero1/1 -> If/2
  [V_GammaError] -> Compare To Zero/1, Compare To Zero1/1
  If/2 -> If Action Subsystem3/Action
  If Action Subsystem/1(Out1) -> Merge/1
  If/3 -> If Action Subsystem1/Action
  [V_GammaAdjustValue] -> If Action Subsystem3/2(In2)
  If Action Subsystem3/1(Out1) -> Merge/2
  If Action Subsystem1/1(Out1) -> Merge/3
  [V_GammaAdjustValue] -> If Action Subsystem/2(In2)
  Compare To Zero/1 -> If/1
  Unit Delay/1 -> [V_LastGammaValue], If Action Subsystem1/1(In1), If Action Subsystem3/1(In1), If Action Subsystem/1(In1)
  If/1 -> If Action Subsystem/Action
  Relational Operator1/1 -> Switch3/2
  [V_GammaError] -> Abs/1
  [V_RampSlope] -> Switch3/1, Relational Operator1/1
  Switch3/1 -> [V_GammaAdjustValue]
  Data Type Conversion4/1 -> Data Type Conversion/1
  Data Type Conversion/1 -> Direct Lookup Table (n-D)1/1
  Add1/1 -> [V_GammaError]
  Abs/1 -> Switch3/3, Relational Operator1/2
  [V_GammaError] -> Compare To Zero2/1
  Compare To Zero2/1 -> V_RampFinished/1

== system Ramp_Library_R2017b/GammaRampLibraryPerLedGroup/RampSlopeCalc ==
  V_RampTime0To100 : Inport
  V_SampleTime : Inport  Port=2
  V_DisableRamp : Inport  Port=3
  Enable : EnablePort
  Compare To Zero : simulink/Logic and Bit Operations/Compare To Zero  relop=~=  OutDataTypeStr=boolean
  Constant : Constant  Value=100  OutMin=0  OutMax=100  OutDataTypeStr=fixdt(0,16,0.01,0)
  If : If  IfExpression=u1 ~= 0
  If Action Subsystem : Subsystem  TreatAsAtomicUnit=on
  If Action Subsystem1 : Subsystem  TreatAsAtomicUnit=on
  Logical Operator : Logic  AllPortsSameDT=off  OutDataTypeStr=boolean
  Logical Operator1 : Logic  Operator=NOT  AllPortsSameDT=off  OutDataTypeStr=boolean
  Merge : Merge  InitialOutput=100
  V_RampSlope : Outport
  wires:
  Logical Operator1/1 -> Logical Operator/2
  V_DisableRamp/1 -> Logical Operator1/1
  Logical Operator/1 -> If/1
  Compare To Zero/1 -> Logical Operator/1
  V_SampleTime/1 -> If Action Subsystem/1(Numerator)
  If/2 -> If Action Subsystem1/Action
  If Action Subsystem1/1(Result) -> Merge/2
  If Action Subsystem/1(Result) -> Merge/1
  Merge/1 -> V_RampSlope/1
  Constant/1 -> If Action Subsystem1/1(DefaultValue)
  V_RampTime0To100/1 -> Compare To Zero/1, If Action Subsystem/2(Denominator)
  If/1 -> If Action Subsystem/Action

== system Ramp_Library_R2017b/GammaRampLibrarySingleLed/If Action Subsystem ==
  In1 : Inport
  In2 : Inport  Port=2
  Action Port : ActionPort
  Add : Sum  OutDataTypeStr=Inherit: Inherit via back propagation
  Out1 : Outport
  wires:
  Add/1 -> Out1/1
  In1/1 -> Add/1
  In2/1 -> Add/2

== system Ramp_Library_R2017b/GammaRampLibrarySingleLed/If Action Subsystem1 ==
  In1 : Inport
  Action Port : ActionPort
  Out1 : Outport
  wires:
  In1/1 -> Out1/1

== system Ramp_Library_R2017b/GammaRampLibrarySingleLed/If Action Subsystem3 ==
  In1 : Inport
  In2 : Inport  Port=2
  Action Port : ActionPort
  Add : Sum  Inputs=+-  OutDataTypeStr=Inherit: Inherit via back propagation
  Out1 : Outport
  wires:
  Add/1 -> Out1/1
  In1/1 -> Add/1
  In2/1 -> Add/2

== system Ramp_Library_R2017b/GammaRampLibrarySingleLed/RampSlopeCalc ==
  V_RampTime0To100 : Inport
  V_SampleTime : Inport  Port=2
  V_DisableRamp : Inport  Port=3
  Enable : EnablePort
  Compare To Zero : simulink/Logic and Bit Operations/Compare To Zero  relop=~=  OutDataTypeStr=boolean
  Constant : Constant  Value=100  OutMin=0  OutMax=100  OutDataTypeStr=fixdt(0,16,0.01,0)
  If : If  IfExpression=u1 ~= 0
  If Action Subsystem : Subsystem  TreatAsAtomicUnit=on
  If Action Subsystem1 : Subsystem  TreatAsAtomicUnit=on
  Logical Operator : Logic  AllPortsSameDT=off  OutDataTypeStr=boolean
  Logical Operator1 : Logic  Operator=NOT  AllPortsSameDT=off  OutDataTypeStr=boolean
  Merge : Merge  InitialOutput=100
  RampSlope : Outport
  wires:
  Logical Operator1/1 -> Logical Operator/2
  V_DisableRamp/1 -> Logical Operator1/1
  Logical Operator/1 -> If/1
  Compare To Zero/1 -> Logical Operator/1
  V_SampleTime/1 -> If Action Subsystem/1(Numerator)
  If/2 -> If Action Subsystem1/Action
  If Action Subsystem1/1(Result) -> Merge/2
  If Action Subsystem/1(Result) -> Merge/1
  Merge/1 -> RampSlope/1
  Constant/1 -> If Action Subsystem1/1(DefaultValue)
  V_RampTime0To100/1 -> Compare To Zero/1, If Action Subsystem/2(Denominator)
  If/1 -> If Action Subsystem/Action

== system Ramp_Library_R2017b/GammaRampLibraryTwoWaysPerLed/If Action Subsystem ==
  In1 : Inport
  In2 : Inport  Port=2
  Action Port : ActionPort
  Add : Sum  OutDataTypeStr=Inherit: Inherit via back propagation
  Out1 : Outport
  wires:
  Add/1 -> Out1/1
  In1/1 -> Add/1
  In2/1 -> Add/2

== system Ramp_Library_R2017b/GammaRampLibraryTwoWaysPerLed/If Action Subsystem1 ==
  In1 : Inport
  Action Port : ActionPort
  Out1 : Outport
  wires:
  In1/1 -> Out1/1

== system Ramp_Library_R2017b/GammaRampLibraryTwoWaysPerLed/If Action Subsystem3 ==
  In1 : Inport
  In2 : Inport  Port=2
  Action Port : ActionPort
  Add : Sum  Inputs=+-  OutDataTypeStr=Inherit: Inherit via back propagation
  Out1 : Outport
  wires:
  Add/1 -> Out1/1
  In1/1 -> Add/1
  In2/1 -> Add/2

== system Ramp_Library_R2017b/GammaRampLibraryTwoWaysPerLed/RampDownSlopeCalc ==
  V_RampTime100To0 : Inport
  V_SampleTime : Inport  Port=2
  V_DisableRamp : Inport  Port=3
  Enable : EnablePort
  Compare To Zero : simulink/Logic and Bit Operations/Compare To Zero  relop=~=  OutDataTypeStr=boolean
  Constant : Constant  Value=100  OutMin=0  OutMax=100  OutDataTypeStr=fixdt(0,16,0.01,0)
  If : If  IfExpression=u1 ~= 0
  If Action Subsystem : Subsystem  TreatAsAtomicUnit=on
  If Action Subsystem1 : Subsystem  TreatAsAtomicUnit=on
  Logical Operator : Logic  AllPortsSameDT=off  OutDataTypeStr=boolean
  Logical Operator1 : Logic  Operator=NOT  AllPortsSameDT=off  OutDataTypeStr=boolean
  Merge : Merge  InitialOutput=100
  V_RampDownSlope : Outport
  wires:
  Logical Operator1/1 -> Logical Operator/2
  V_DisableRamp/1 -> Logical Operator1/1
  Logical Operator/1 -> If/1
  Compare To Zero/1 -> Logical Operator/1
  V_SampleTime/1 -> If Action Subsystem/1(Numerator)
  If/2 -> If Action Subsystem1/Action
  If Action Subsystem1/1(Result) -> Merge/2
  If Action Subsystem/1(Result) -> Merge/1
  Merge/1 -> V_RampDownSlope/1
  Constant/1 -> If Action Subsystem1/1(DefaultValue)
  V_RampTime100To0/1 -> Compare To Zero/1, If Action Subsystem/2(Denominator)
  If/1 -> If Action Subsystem/Action

== system Ramp_Library_R2017b/GammaRampLibraryTwoWaysPerLed/RampUpSlopeCalc ==
  V_RampTime0To100 : Inport
  V_SampleTime : Inport  Port=2
  V_DisableRamp : Inport  Port=3
  Enable : EnablePort
  Compare To Zero : simulink/Logic and Bit Operations/Compare To Zero  relop=~=  OutDataTypeStr=boolean
  Constant : Constant  Value=100  OutMin=0  OutMax=100  OutDataTypeStr=fixdt(0,16,0.01,0)
  If : If  IfExpression=u1 ~= 0
  If Action Subsystem : Subsystem  TreatAsAtomicUnit=on
  If Action Subsystem1 : Subsystem  TreatAsAtomicUnit=on
  Logical Operator : Logic  AllPortsSameDT=off  OutDataTypeStr=boolean
  Logical Operator1 : Logic  Operator=NOT  AllPortsSameDT=off  OutDataTypeStr=boolean
  Merge : Merge  InitialOutput=100
  V_RampUpSlope : Outport
  wires:
  If/1 -> If Action Subsystem/Action
  V_RampTime0To100/1 -> If Action Subsystem/2(Denominator), Compare To Zero/1
  Constant/1 -> If Action Subsystem1/1(DefaultValue)
  Merge/1 -> V_RampUpSlope/1
  If Action Subsystem/1(Result) -> Merge/1
  If Action Subsystem1/1(Result) -> Merge/2
  If/2 -> If Action Subsystem1/Action
  V_SampleTime/1 -> If Action Subsystem/1(Numerator)
  Compare To Zero/1 -> Logical Operator/1
  Logical Operator/1 -> If/1
  V_DisableRamp/1 -> Logical Operator1/1
  Logical Operator1/1 -> Logical Operator/2

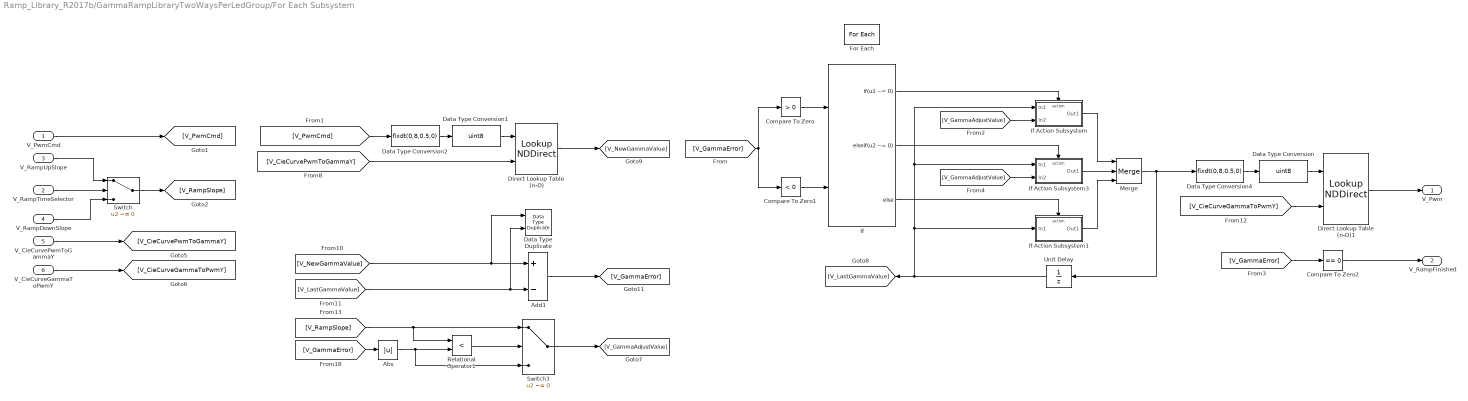
== system Ramp_Library_R2017b/GammaRampLibraryTwoWaysPerLedGroup/For Each Subsystem ==
  V_PwmCmd : Inport  Partition=on  PartitionDimension=1  PartitionWidth=1  PartitionOffset=0
  V_RampTimeSelector : Inport  Port=2  Partition=on  PartitionDimension=1  PartitionWidth=1  PartitionOffset=0
  V_RampUpSlope : Inport  Port=3
  V_RampDownSlope : Inport  Port=4
  V_CieCurvePwmToGammaY : Inport  Port=5
  V_CieCurveGammaToPwmY : Inport  Port=6
  Abs : Abs
  Add1 : Sum  Inputs=+-  OutMin=-100  OutMax=100  OutDataTypeStr=fixdt(1,16,0.01,0)
  Compare To Zero : simulink/Logic and Bit Operations/Compare To Zero  relop=>  OutDataTypeStr=boolean
  Compare To Zero1 : simulink/Logic and Bit Operations/Compare To Zero  relop=<  OutDataTypeStr=boolean
  Compare To Zero2 : simulink/Logic and Bit Operations/Compare To Zero  relop===  OutDataTypeStr=boolean
  Data Type Duplicate : DataTypeDuplicate
  Data Type Conversion : DataTypeConversion  OutDataTypeStr=uint8  ConvertRealWorld=Stored Integer (SI)
  Data Type Conversion1 : DataTypeConversion  OutDataTypeStr=uint8  ConvertRealWorld=Stored Integer (SI)
  Data Type Conversion2 : DataTypeConversion  OutDataTypeStr=fixdt(0,8,0.5,0)  RndMeth=Round
  Data Type Conversion4 : DataTypeConversion  OutDataTypeStr=fixdt(0,8,0.5,0)  RndMeth=Round
  Direct Lookup Table (n-D) : LookupNDDirect  NumberOfTableDimensions=1  TableIsInput=on
  Direct Lookup Table (n-D)1 : LookupNDDirect  NumberOfTableDimensions=1  TableIsInput=on
  For Each : ForEach  DisableCoverage=on  IndexMode=One-based
  If : If  NumInputs=2  IfExpression=u1 ~= 0  ElseIfExpressions=u2 ~= 0
  If Action Subsystem : Subsystem  TreatAsAtomicUnit=on
  If Action Subsystem1 : Subsystem  TreatAsAtomicUnit=on
  If Action Subsystem3 : Subsystem  TreatAsAtomicUnit=on
  Merge : Merge  Inputs=3
  Relational Operator1 : RelationalOperator  Operator=<  OutDataTypeStr=boolean  RndMeth=Simplest
  Switch : Switch  Criteria=u2 ~= 0
  Switch3 : Switch  Criteria=u2 ~= 0  OutDataTypeStr=Inherit: Inherit via back propagation
  Unit Delay : UnitDelay  SampleTime=-1
  V_Pwm : Outport  ConcatenationDimension=1
  V_RampFinished : Outport  Port=2  ConcatenationDimension=1
  wires:
  Compare To Zero2/1 -> V_RampFinished/1
  [V_GammaError] -> Compare To Zero2/1
  Abs/1 -> Relational Operator1/2, Switch3/3
  Add1/1 -> [V_GammaError]
  Data Type Conversion/1 -> Direct Lookup Table (n-D)1/1
  Data Type Conversion4/1 -> Data Type Conversion/1
  Switch3/1 -> [V_GammaAdjustValue]
  [V_RampSlope] -> Relational Operator1/1, Switch3/1
  [V_GammaError] -> Abs/1
  Relational Operator1/1 -> Switch3/2
  If/1 -> If Action Subsystem/Action
  Unit Delay/1 -> If Action Subsystem/1(In1), If Action Subsystem3/1(In1), If Action Subsystem1/1(In1), [V_LastGammaValue]
  Compare To Zero/1 -> If/1
  [V_GammaAdjustValue] -> If Action Subsystem/2(In2)
  If Action Subsystem1/1(Out1) -> Merge/3
  If Action Subsystem3/1(Out1) -> Merge/2
  [V_GammaAdjustValue] -> If Action Subsystem3/2(In2)
  If/3 -> If Action Subsystem1/Action
  If Action Subsystem/1(Out1) -> Merge/1
  If/2 -> If Action Subsystem3/Action
  [V_GammaError] -> Compare To Zero1/1, Compare To Zero/1
  Compare To Zero1/1 -> If/2
  Data Type Conversion1/1 -> Direct Lookup Table (n-D)/1
  Merge/1 -> Unit Delay/1, Data Type Conversion4/1
  [V_CieCurveGammaToPwmY] -> Direct Lookup Table (n-D)1/2
  [V_LastGammaValue] -> Add1/2, Data Type Duplicate/2
  [V_NewGammaValue] -> Add1/1, Data Type Duplicate/1
  Direct Lookup Table (n-D)1/1 -> V_Pwm/1
  [V_CieCurvePwmToGammaY] -> Direct Lookup Table (n-D)/2
  Data Type Conversion2/1 -> Data Type Conversion1/1
  V_RampUpSlope/1 -> Switch/1
  V_CieCurvePwmToGammaY/1 -> [V_CieCurvePwmToGammaY]
  V_CieCurveGammaToPwmY/1 -> [V_CieCurveGammaToPwmY]
  V_PwmCmd/1 -> [V_PwmCmd]
  Direct Lookup Table (n-D)/1 -> [V_NewGammaValue]
  [V_PwmCmd] -> Data Type Conversion2/1
  V_RampTimeSelector/1 -> Switch/2
  Switch/1 -> [V_RampSlope]
  V_RampDownSlope/1 -> Switch/3

== system Ramp_Library_R2017b/GammaRampLibraryTwoWaysPerLedGroup/RampDownSlopeCalc ==
  V_RampTime100To0 : Inport
  V_SampleTime : Inport  Port=2
  V_DisableRamp : Inport  Port=3
  Enable : EnablePort
  Compare To Zero : simulink/Logic and Bit Operations/Compare To Zero  relop=~=  OutDataTypeStr=boolean
  Constant : Constant  Value=100  OutMin=0  OutMax=100  OutDataTypeStr=fixdt(0,16,0.01,0)
  If : If  IfExpression=u1 ~= 0
  If Action Subsystem : Subsystem  TreatAsAtomicUnit=on
  If Action Subsystem1 : Subsystem  TreatAsAtomicUnit=on
  Logical Operator : Logic  AllPortsSameDT=off  OutDataTypeStr=boolean
  Logical Operator1 : Logic  Operator=NOT  AllPortsSameDT=off  OutDataTypeStr=boolean
  Merge : Merge  InitialOutput=100
  V_RampDownSlope : Outport
  wires:
  Logical Operator1/1 -> Logical Operator/2
  V_DisableRamp/1 -> Logical Operator1/1
  Logical Operator/1 -> If/1
  Compare To Zero/1 -> Logical Operator/1
  V_SampleTime/1 -> If Action Subsystem/1(Numerator)
  If/2 -> If Action Subsystem1/Action
  If Action Subsystem1/1(Result) -> Merge/2
  If Action Subsystem/1(Result) -> Merge/1
  Merge/1 -> V_RampDownSlope/1
  Constant/1 -> If Action Subsystem1/1(DefaultValue)
  V_RampTime100To0/1 -> Compare To Zero/1, If Action Subsystem/2(Denominator)
  If/1 -> If Action Subsystem/Action

== system Ramp_Library_R2017b/GammaRampLibraryTwoWaysPerLedGroup/RampUpSlopeCalc ==
  V_RampTime0To100 : Inport
  V_SampleTime : Inport  Port=2
  V_DisableRamp : Inport  Port=3
  Enable : EnablePort
  Compare To Zero : simulink/Logic and Bit Operations/Compare To Zero  relop=~=  OutDataTypeStr=boolean
  Constant : Constant  Value=100  OutMin=0  OutMax=100  OutDataTypeStr=fixdt(0,16,0.01,0)
  If : If  IfExpression=u1 ~= 0
  If Action Subsystem : Subsystem  TreatAsAtomicUnit=on
  If Action Subsystem1 : Subsystem  TreatAsAtomicUnit=on
  Logical Operator : Logic  AllPortsSameDT=off  OutDataTypeStr=boolean
  Logical Operator1 : Logic  Operator=NOT  AllPortsSameDT=off  OutDataTypeStr=boolean
  Merge : Merge  InitialOutput=100
  V_RampUpSlope : Outport
  wires:
  If/1 -> If Action Subsystem/Action
  V_RampTime0To100/1 -> If Action Subsystem/2(Denominator), Compare To Zero/1
  Constant/1 -> If Action Subsystem1/1(DefaultValue)
  Merge/1 -> V_RampUpSlope/1
  If Action Subsystem/1(Result) -> Merge/1
  If Action Subsystem1/1(Result) -> Merge/2
  If/2 -> If Action Subsystem1/Action
  V_SampleTime/1 -> If Action Subsystem/1(Numerator)
  Compare To Zero/1 -> Logical Operator/1
  Logical Operator/1 -> If/1
  V_DisableRamp/1 -> Logical Operator1/1
  Logical Operator1/1 -> Logical Operator/2
